simulink model "Figure_3_3_TP_ModulationFrequencePorteuse"  (R2020a)
settings: Solver=VariableStepAuto  StartTime=0.0  StopTime=10.0  RelTol=1e-3
model workspace (MAT data in the model file):
  K = Simulink.Parameter
  K.DataType = 'auto'
  K.Dimensions = [0 0]
libraries: commdigbbndam3 x4, commchan3 x1, commsink2 x1, commrandsrc3 x1
settings Model: Creator=iba  LastModifiedBy=iba

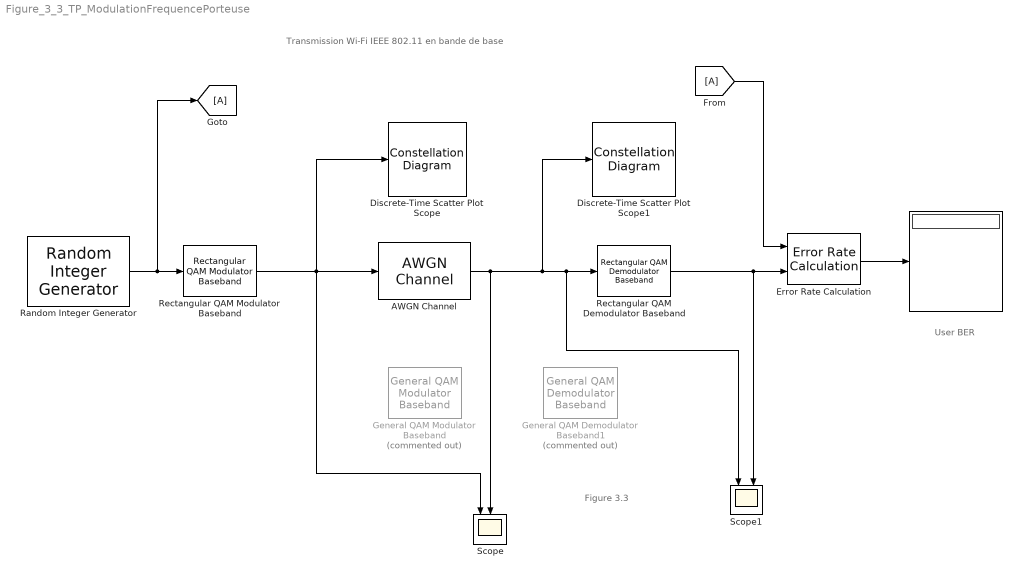
== system Figure_3_3_TP_ModulationFrequencePorteuse ==
  note: User BER
  note: Figure 3.3
  note: Transmission Wi-Fi IEEE 802.11 en bande de base
  " " : Display
  AWGN Channel : commchan3/AWGN Channel  InputProcessing=Columns as channels (frame based)  seed=1  noiseMode="Signal to noise ratio  (SNR)"  EbNodB=15  EsNodB=10  SNRdB=100  bitsPerSym=1  Ps=100  Tsym=10  variance=1
  Discrete-Time Scatter Plot Scope : ConstellationDiagram
  Discrete-Time Scatter Plot Scope1 : ConstellationDiagram
  "Error Rate Calculation " : commsink2/Error Rate Calculation  N=1  st_delay=0  cp_mode=Entire frame  subframe=[]  PMode=Port  WsName=ErrorVec  RsMode2=off  stop=off  numErr=100  maxBits=1e6
  "General QAM Demodulator Baseband1 " : commdigbbndam3/General QAM Demodulator Baseband  Commented=on  SigCon=[exp(2*pi*1i*[0:7]/8)]  OutType=Integer  DecType=Hard decision  VarSource=Dialog  Variance=1  outDtypeBit=Inherit via internal rule  outDtype=Inherit via internal rule  roundingMode=Floor  overflowMode=Wrap  OvFlMode=off  OvFlModeLastStrValue=off  sigConstWordLen=16  sigConstDataTypeStr=Inherit: Same word length as input  sigConstLastDataTypeStr=Inherit: Same word length as input  accum1WordLen=32  accum1FracLen=30  prodInWordLen=32  prodInFracLen=30  prodInDataTypeStr=Inherit: Same as accumulator 1  prodInLastDataTypeStr=Inherit: Same as accumulator 1  prodOutWordLen=32  prodOutFracLen=30  accum2WordLen=32  accum2FracLen=30  accum3WordLen=32  accum3FracLen=30  nsiWordLen=32  nsiFracLen=30  nsiDataTypeStr=Inherit: Same as accumulator 3  nsiLastDataTypeStr=Inherit: Same as accumulator 3  invn0WordLen=16  invn0FracLen=8  invn0DataTypeStr=Inherit: Same word length as input  invn0LastDataTypeStr=Inherit: Same word length as input  outputWordLen=32  outputFracLen=30
      settings: SourceProductBaseCode=CM
  "General QAM Modulator Baseband " : commdigbbndam3/General QAM Modulator Baseband  Commented=on  SigCon=[exp(2*pi*1i*[0:7]/8)]  outDtype=double  outWordLen=16  outUDDataType=sfix(16)  outFracLenMode=Best precision  outFracLen=15  outDataTypeStr=double  outLastDataTypeStr=double
      settings: SourceProductBaseCode=CM
  "Random Integer Generator " : commrandsrc3/Random Integer Generator  SetSize=4  SeedSource=Parameter  Seed=0  SampleTime=0.01  SamplesPerFrame=1  OutputDataType=double  SimulateUsing=Interpreted execution
  "Rectangular QAM Demodulator Baseband " : commdigbbndam3/Rectangular QAM Demodulator Baseband  M=64  OutType=Integer  DecType=Hard decision  VarSource=Dialog  Variance=1  Dec=Gray  Mapping=[0:15]  PowType=Peak Power  MinDist=0.1  AvgPow=1  PeakPow=0.01  Ph=0  outDtype1=Inherit via internal rule  outDtype2=Inherit via internal rule  derotateFactorWordLen=16  derotateFactorDataTypeStr=Inherit: Same word length as input  derotateFactorLastDataTypeStr=Inherit: Same word length as input  denormFactorWordLen=16  denormFactorDataTypeStr=Inherit: Same word length as input  denormFactorLastDataTypeStr=Inherit: Same word length as input  prodOutWordLen=32  prodOutOverflowMode=Wrap  prodOutRoundingMode=Floor  prodOutOvFlMode=off  prodOutOvFlModeLastStrValue=off  sumWordLen=32
  "Rectangular QAM Modulator Baseband " : commdigbbndam3/Rectangular QAM Modulator Baseband  M=64  InType=Integer  Enc=Gray  Mapping=[0:15]  PowType=Min. distance between symbols  MinDist=0.1  AvgPow=1  PeakPow=1  Ph=0  outDtype=double  outWordLen=16  outUDDataType=sfix(16)  outFracLenMode=Best precision  outFracLen=15  outDataTypeStr=double  outLastDataTypeStr=double
  Scope : Scope  NumInputPorts=3
  Scope1 : Scope  NumInputPorts=2
  wires:
  "Rectangular QAM Modulator Baseband "/1 -> Scope/1, AWGN Channel/1, Discrete-Time Scatter Plot Scope/1
  "Random Integer Generator "/1 -> [A], "Rectangular QAM Modulator Baseband "/1
  "Error Rate Calculation "/1 -> " "/1
  AWGN Channel/1 -> Scope1/1, "Rectangular QAM Demodulator Baseband "/1, Discrete-Time Scatter Plot Scope1/1, Scope/2
  "Rectangular QAM Demodulator Baseband "/1 -> Scope1/2, "Error Rate Calculation "/2
  [A] -> "Error Rate Calculation "/1
